simulink model "model"  (Simulink 7.5)
settings: Solver=ode1  StartTime=0.0  StopTime=czas_sym  FixedStep=ts  RelTol=1e-3
undefined symbols (not defined in the file): f, i, ksi, limit, lr, wi_init, wo_init, wr, wz
libraries: neural x1
settings Model: Creator=ja  LastModifiedBy=Hubert
settings OptimizationCC: InitFltsAndDblsToZero=on
settings DebuggingCC: StrictBusMsg=Warning

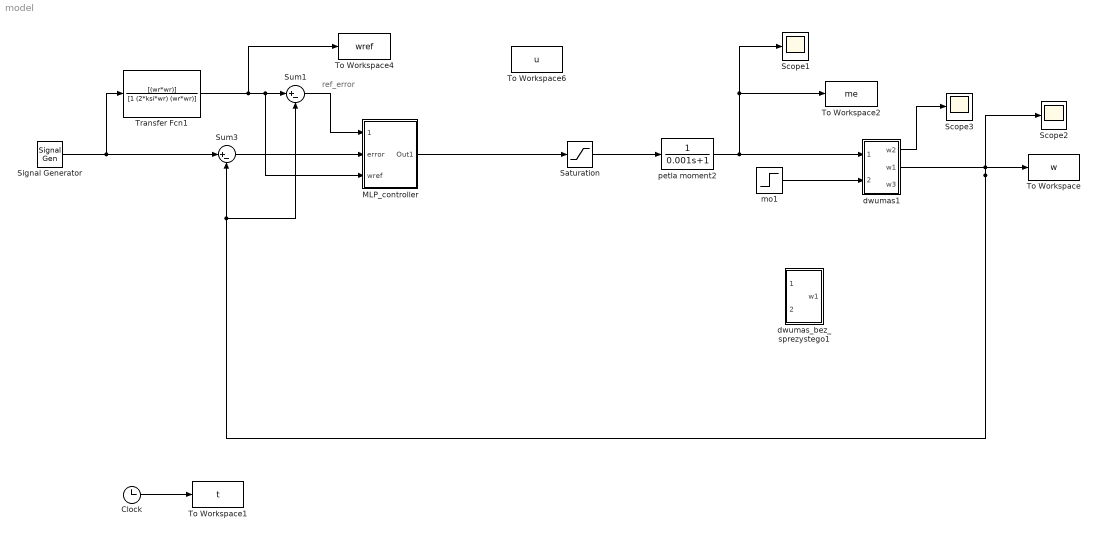
== system model ==
  note: ref_error
  Clock : Clock
      settings: Decimation=10
  MLP_controller : Subsystem
  Saturation : Saturate  UpperLimit=limit  LowerLimit=-limit  OutDataType=sfix(16)  OutScaling=2^0
  Scope1 : Scope
      settings: TimeRange=5  YMin=-8e+071  YMax=1e+071
  Scope2 : Scope
      settings: TimeRange=5  YMin=-0.275  YMax=0.3
  Scope3 : Scope
      settings: TimeRange=5  YMin=-0.275  YMax=0.3  SaveName=ScopeData2
  Signal Generator : SignalGenerator  WaveForm=square  Amplitude=wz  Frequency=f
  Sum1 : Sum  Inputs=|+-  SaturateOnIntegerOverflow=on  InputSameDT=on  OutDataTypeStr=Inherit: Same as first input
  Sum3 : Sum  Inputs=|+-  SaturateOnIntegerOverflow=on  InputSameDT=on  OutDataTypeStr=Inherit: Same as first input
  To Workspace : ToWorkspace  VariableName=w  SampleTime=-1  SaveFormat=Array
  To Workspace1 : ToWorkspace  VariableName=t  SampleTime=-1  SaveFormat=Array
  To Workspace2 : ToWorkspace  VariableName=me  SampleTime=-1  SaveFormat=Array
  To Workspace4 : ToWorkspace  VariableName=wref  SampleTime=-1  SaveFormat=Array
  To Workspace6 : ToWorkspace  VariableName=u  SampleTime=-1  SaveFormat=Array
  Transfer Fcn1 : TransferFcn  Numerator=[(wr*wr)]  Denominator=[1 (2*ksi*wr) (wr*wr)]
  dwumas1 : Subsystem
  dwumas_bez_sprezystego1 : Subsystem
  mo1 : Step  Time=3.6  SampleTime=0
  petla moment2 : TransferFcn  Denominator=[0.001 1]
  wires:
  petla moment2/1 -> Scope1/1, To Workspace2/1, dwumas1/1(me)
  Signal Generator/1 -> Transfer Fcn1/1, Sum3/1
  Saturation/1 -> petla moment2/1
  Sum3/1 -> MLP_controller/2(error)
  dwumas1/2(w1) -> Scope2/1, Sum3/2, Sum1/2, To Workspace/1
  Clock/1 -> To Workspace1/1
  mo1/1 -> dwumas1/2(mo)
  Transfer Fcn1/1 -> To Workspace4/1, Sum1/1, MLP_controller/3(wref)
  Sum1/1 -> MLP_controller/1(ref_error)
  dwumas1/1(w2) -> Scope3/1
  MLP_controller/1(Out1) -> Saturation/1

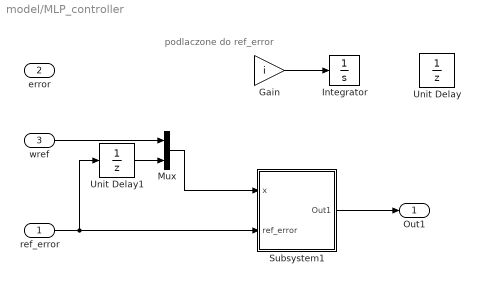
== system model/MLP_controller ==
  note: podlaczone do ref_error
  ref_error : Inport
  error : Inport  Port=2
  wref : Inport  Port=3
  Gain : Gain  Gain=i  ParameterDataType=fixdt(1, 16)  ParameterScaling=2^0  OutDataType=fixdt(1, 16)  OutScaling=2^0
  Integrator : Integrator
  Mux : Mux  Inputs=2
  Subsystem1 : Subsystem
  Unit Delay : UnitDelay  SampleTime=-1
  Unit Delay1 : UnitDelay  SampleTime=-1
  Out1 : Outport
  wires:
  Mux/1 -> Subsystem1/1(x)
  Subsystem1/1(Out1) -> Out1/1
  ref_error/1 -> Subsystem1/2(ref_error), Unit Delay1/1
  Gain/1 -> Integrator/1
  wref/1 -> Mux/1
  Unit Delay1/1 -> Mux/2

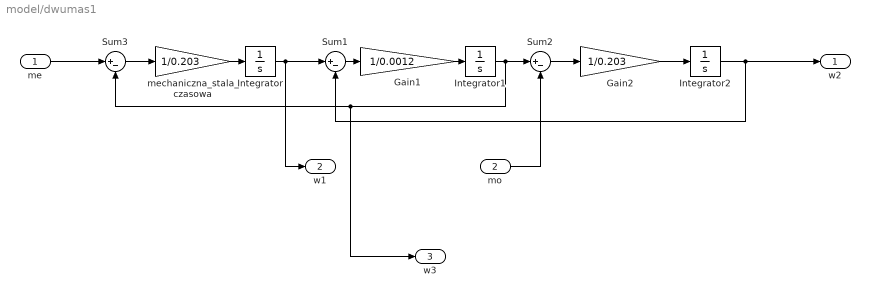
== system model/dwumas1 ==
  me : Inport
  mo : Inport  Port=2
  Gain1 : Gain  Gain=1/0.0012  ParameterDataType=fixdt(1, 16)  ParameterScaling=2^0  OutDataType=fixdt(1, 16)  OutScaling=2^0
  Gain2 : Gain  Gain=1/0.203  ParameterDataType=fixdt(1, 16)  ParameterScaling=2^0  OutDataType=fixdt(1, 16)  OutScaling=2^0
  Integrator : Integrator
  Integrator1 : Integrator
  Integrator2 : Integrator
  Sum1 : Sum  Inputs=|+-  OutDataType=fixdt(1, 16)  OutScaling=2^0
  Sum2 : Sum  Inputs=|+-  OutDataType=fixdt(1, 16)  OutScaling=2^0
  Sum3 : Sum  Inputs=|+-  OutDataType=fixdt(1, 16)  OutScaling=2^0
  mechaniczna_stala_czasowa : Gain  Gain=1/0.203  ParameterDataType=fixdt(1, 16)  ParameterScaling=2^0  OutDataType=fixdt(1, 16)  OutScaling=2^0
  w2 : Outport  OutDataType=fixdt(1, 16)  OutScaling=2^0
  w1 : Outport  Port=2  OutDataType=fixdt(1, 16)  OutScaling=2^0
  w3 : Outport  Port=3  OutDataType=fixdt(1, 16)  OutScaling=2^0
  wires:
  mechaniczna_stala_czasowa/1 -> Integrator/1
  Integrator/1 -> Sum1/1, w1/1
  Sum3/1 -> mechaniczna_stala_czasowa/1
  Integrator1/1 -> Sum2/1, Sum3/2, w3/1
  Gain1/1 -> Integrator1/1
  Sum1/1 -> Gain1/1
  Sum2/1 -> Gain2/1
  Gain2/1 -> Integrator2/1
  Integrator2/1 -> Sum1/2, w2/1
  me/1 -> Sum3/1
  mo/1 -> Sum2/2

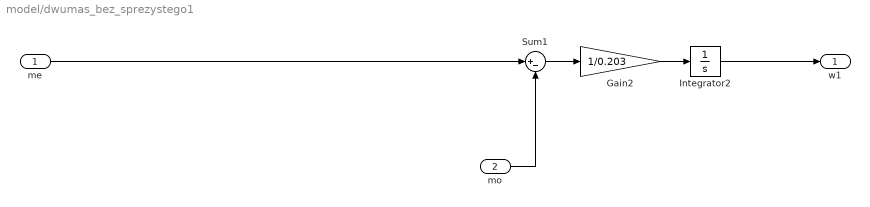
== system model/dwumas_bez_sprezystego1 ==
  me : Inport
  mo : Inport  Port=2
  Gain2 : Gain  Gain=1/0.203  ParameterDataType=fixdt(1, 16)  ParameterScaling=2^0  OutDataType=fixdt(1, 16)  OutScaling=2^0
  Integrator2 : Integrator
  Sum1 : Sum  Inputs=|+-  OutDataType=fixdt(1, 16)  OutScaling=2^0
  w1 : Outport  OutDataType=fixdt(1, 16)  OutScaling=2^0
  wires:
  Integrator2/1 -> w1/1
  Gain2/1 -> Integrator2/1
  Sum1/1 -> Gain2/1
  mo/1 -> Sum1/2
  me/1 -> Sum1/1

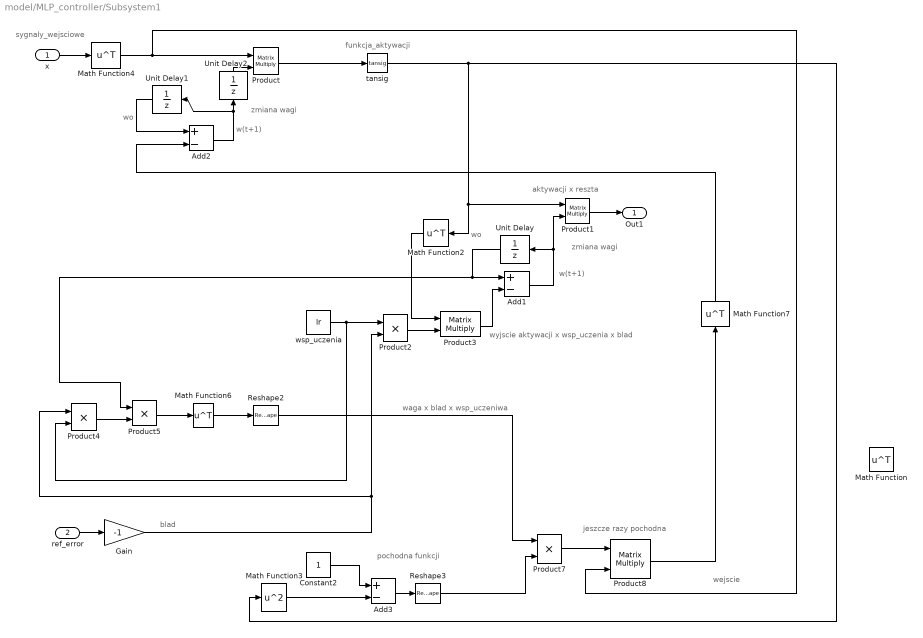
== system model/MLP_controller/Subsystem1 ==
  note: wo
  note: funkcja_aktywacji
  note: blad
  note: pochodna funkcji
  note: w(t+1)
  note: wo
  note: w(t+1)
  note: sygnaly_wejsciowe
  note: zmiana wagi
  note: zmiana wagi
  note: waga x blad x wsp_uczeniwa
  note: jeszcze razy pochodna
  note: wejscie
  note: wyjscie aktywacji x wsp_uczenia x blad
  note: aktywacji x reszta
  x : Inport  OutDataType=sfix(16)  OutScaling=2^0
  ref_error : Inport  Port=2  OutDataType=sfix(16)  OutScaling=2^0
  Add1 : Sum  Inputs=+-  OutDataType=sfix(16)  OutScaling=2^-10
  Add2 : Sum  Inputs=+-  OutDataType=sfix(16)  OutScaling=2^-10
  Add3 : Sum  Inputs=+-  OutDataType=sfix(16)  OutScaling=2^-10
  Constant2 : Constant  OutDataType=sfix(16)  OutScaling=2^0
  Gain : Gain  Gain=-1  ParameterDataType=fixdt(1, 16)  ParameterScaling=2^0  OutDataType=fixdt(1, 16)  OutScaling=2^0
  Math Function : Math  Operator=transpose  OutDataType=fixdt(1, 16)  OutScaling=2^0  SaturateOnIntegerOverflow=on
  Math Function{2,4,6..7} (4 alike) : Math  Operator=transpose  OutDataType=sfix(16)  OutScaling=2^0  SaturateOnIntegerOverflow=on
  Math Function3 : Math  Operator=square  OutDataType=sfix(16)  OutScaling=2^0  SaturateOnIntegerOverflow=on
  Product{,1,3,8} (4 alike) : Product  Multiplication=Matrix(*)  OutDataType=sfix(16)  OutScaling=2^0  RndMeth=Zero
  Product{2,4..5,7} (4 alike) : Product  OutDataType=sfix(16)  OutScaling=2^0  RndMeth=Zero
  Reshape2 : Reshape  OutputDimensionality=Column vector (2-D)
  Reshape3 : Reshape  OutputDimensionality=Column vector (2-D)
  Unit Delay : UnitDelay  X0=wo_init  SampleTime=-1
  Unit Delay1 : UnitDelay  X0=wi_init  SampleTime=-1
  Unit Delay2 : UnitDelay  X0=wi_init  SampleTime=-1
  tansig : neural/Transfer Functions/tansig  SystemSampleTime=-1
  wsp_uczenia : Constant  Value=lr  OutDataType=sfix(16)  OutScaling=2^0
  Out1 : Outport  OutDataType=sfix(16)  OutScaling=2^0
  wires:
  Add2/1 -> Unit Delay1/1, Unit Delay2/1
  Product8/1 -> Math Function7/1
  Reshape3/1 -> Product7/2
  Reshape2/1 -> Product7/1
  Math Function3/1 -> Add3/2
  Constant2/1 -> Add3/1
  Product4/1 -> Product5/2
  Math Function2/1 -> Product3/1
  Product2/1 -> Product3/2
  wsp_uczenia/1 -> Product2/1, Product4/2
  Product1/1 -> Out1/1
  tansig/1 -> Product1/1, Math Function2/1, Math Function3/1
  Product/1 -> tansig/1
  Add3/1 -> Reshape3/1
  Product5/1 -> Math Function6/1
  Math Function6/1 -> Reshape2/1
  Math Function4/1 -> Product/1, Product8/2
  x/1 -> Math Function4/1
  ref_error/1 -> Gain/1
  Gain/1 -> Product2/2, Product4/1
  Unit Delay1/1 -> Add2/1
  Unit Delay/1 -> Add1/1, Product5/1
  Add1/1 -> Product1/2, Unit Delay/1
  Product3/1 -> Add1/2
  Math Function7/1 -> Add2/2
  Product7/1 -> Product8/1
  Unit Delay2/1 -> Product/2
